simulink model "REALTIME_PARTBONUS_extended"  (R2020b)
settings: Solver=ode3  StartTime=0.0  StopTime=5  FixedStep=0.001  RelTol=1e-3
undefined symbols (not defined in the file): Aest, Ar, Best, Cest, Dest, K3, National_Instruments, PCI, rads2rpm, rpm2rads, sens, Tr
libraries: sldrtlib x2
settings Model: ExtModeTrigDuration=10000  Creator=utente  LastModifiedBy=ambrosingi
settings DataIOCC: ReturnWorkspaceOutputs=off
settings RTWCC: Description=Simulink Desktop Real-Time  SystemTargetFile=sldrt.tlc  TemplateMakefile=sldrt.tmf  RTWCompilerOptimization=on
settings CodeAppCC: MaxIdLength=95
settings SimulinkDesktopRealTimeCC: TargetPreCompLibLocation=C:\Program Files\MATLAB\R2020b\toolbox\sldrt\lib\win64

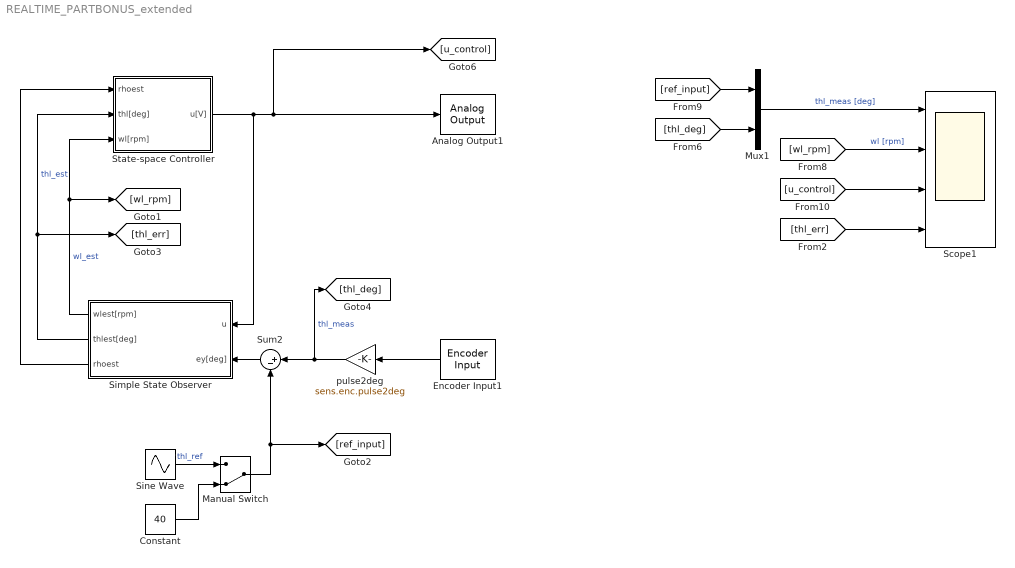
== system REALTIME_PARTBONUS_extended ==
  Analog Output1 : sldrtlib/Analog Output  SampleTime=0.001  MaxMissedTicks=10  ShowMissedTicks=off  YieldWhenWaiting=off  DrvName=National_Instruments/PCI-6221  DrvAddress=4294967295  DrvOptions=[0 0 0 2 0]  Channels=1  RangeMode=1  VoltRange=1  InitialValue=0  FinalValue=0
      settings: AttributesFormatString=National Instruments\nPCI-6221 [auto]
  Constant : Constant  Value=40
  Encoder Input1 : sldrtlib/Encoder Input  SampleTime=0.001  MaxMissedTicks=10  ShowMissedTicks=off  YieldWhenWaiting=off  DrvName=National_Instruments/PCI-6221  DrvAddress=4294967295  DrvOptions=[0 0 0 2 0]  Channels=1  QuadMode=3  IndexPulse=1  InputFilter=Inf  DataType=1
      settings: AttributesFormatString=National Instruments\nPCI-6221 [auto]
  Manual Switch : ManualSwitch  CurrentSetting=0
  Mux1 : Mux  Inputs=2
  Scope1 : Scope  NumInputPorts=4
  Simple State Observer : Subsystem
  Sine Wave : Sin  Amplitude=Ar  Frequency=2*pi/Tr  SampleTime=0
  State-space Controller : Subsystem
  Sum2 : Sum  Inputs=|+-
  pulse2deg : Gain  Gain=sens.enc.pulse2deg
  wires:
  Encoder Input1/1 -> pulse2deg/1
  Sum2/1 -> Simple State Observer/2(ey[deg])
  pulse2deg/1 -> [thl_deg], Sum2/1  "thl_meas"
  Simple State Observer/3(rhoest) -> State-space Controller/1(rhoest)
  Simple State Observer/2(thlest[deg]) -> [thl_err], State-space Controller/2(thl[deg])  "thl_est"
  Simple State Observer/1(wlest[rpm]) -> [wl_rpm], State-space Controller/3(wl[rpm])  "wl_est"
  Sine Wave/1 -> Manual Switch/1  "thl_ref"
  Constant/1 -> Manual Switch/2
  Manual Switch/1 -> [ref_input], Sum2/2
  [ref_input] -> Mux1/1
  [wl_rpm] -> Scope1/2  "wl [rpm]"
  [thl_deg] -> Mux1/2
  Mux1/1 -> Scope1/1  "thl_meas [deg]"
  State-space Controller/1(u[V]) -> [u_control], Analog Output1/1, Simple State Observer/1(u)
  [u_control] -> Scope1/3
  [thl_err] -> Scope1/4

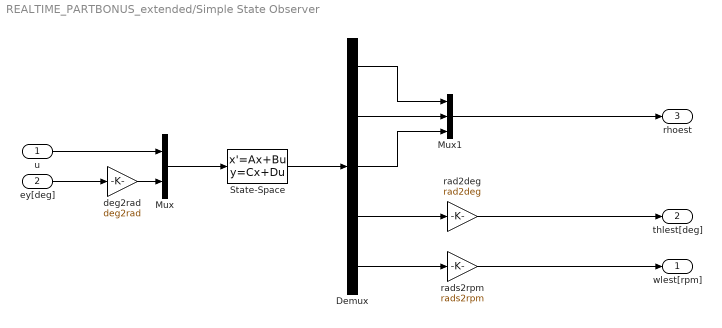
== system REALTIME_PARTBONUS_extended/Simple State Observer ==
  u : Inport
  ey[deg] : Inport  Port=2
  Demux : Demux  Outputs=5
  Mux : Mux  Inputs=2
  Mux1 : Mux  Inputs=3
  State-Space : StateSpace  A=Aest  B=Best  C=Cest  D=Dest  InitialCondition=0
  deg2rad : Gain  Gain=deg2rad
  rad2deg : Gain  Gain=rad2deg
  rads2rpm : Gain  Gain=rads2rpm
  wlest[rpm] : Outport
  thlest[deg] : Outport  Port=2
  rhoest : Outport  Port=3
  wires:
  Mux/1 -> State-Space/1
  State-Space/1 -> Demux/1
  ey[deg]/1 -> deg2rad/1
  u/1 -> Mux/1
  Demux/1 -> Mux1/1
  Demux/2 -> Mux1/2
  Demux/3 -> Mux1/3
  Mux1/1 -> rhoest/1
  Demux/4 -> rad2deg/1
  rads2rpm/1 -> wlest[rpm]/1
  Demux/5 -> rads2rpm/1
  rad2deg/1 -> thlest[deg]/1
  deg2rad/1 -> Mux/2

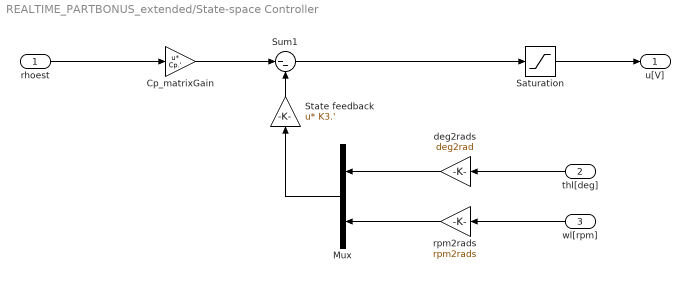
== system REALTIME_PARTBONUS_extended/State-space Controller ==
  rhoest : Inport
  thl[deg] : Inport  Port=2
  wl[rpm] : Inport  Port=3
  Cp_matrixGain : Gain  Gain=Cp.'  Multiplication=Matrix(u*K)
  Mux : Mux  Inputs=2
  Saturation : Saturate  UpperLimit=10  LowerLimit=-10
  State feedback : Gain  Gain=K3.'  Multiplication=Matrix(u*K)
  Sum1 : Sum  Inputs=|--
  deg2rads : Gain  Gain=deg2rad
  rpm2rads : Gain  Gain=rpm2rads
  u[V] : Outport
  wires:
  Saturation/1 -> u[V]/1
  deg2rads/1 -> Mux/1
  rpm2rads/1 -> Mux/2
  thl[deg]/1 -> deg2rads/1
  wl[rpm]/1 -> rpm2rads/1
  Mux/1 -> State feedback/1
  rhoest/1 -> Cp_matrixGain/1
  State feedback/1 -> Sum1/2
  Cp_matrixGain/1 -> Sum1/1
  Sum1/1 -> Saturation/1
